simulink model "SimulinkController"  (R2016b)
settings: Solver=VariableStepAuto  StartTime=0.0  StopTime=40.0  RelTol=1e-3
undefined symbols (not defined in the file): K
settings Model: Creator=kwstas  LastModifiedBy=kwstas
settings SolverCC: MaxConsecutiveZCs=10000

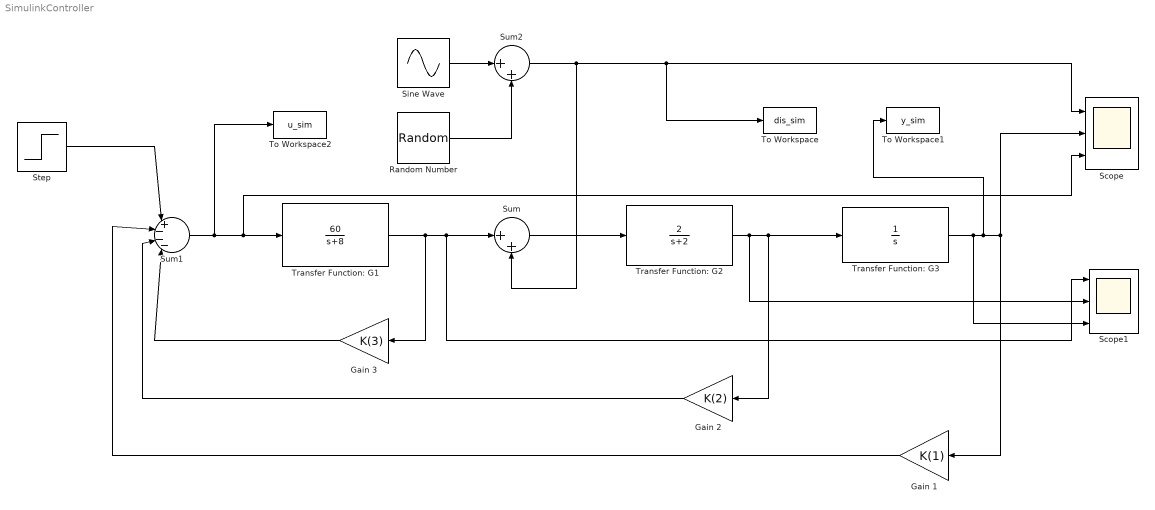
== system SimulinkController ==
  Gain 1 : Gain  Gain=K(1)
  "Gain 2 " : Gain  Gain=K(2)
  "Gain 3 " : Gain  Gain=K(3)
  Random Number : RandomNumber  Variance=5  SampleTime=0.1
  Scope : Scope  NumInputPorts=3
  Scope1 : Scope  NumInputPorts=3
  Sine Wave : Sin  Frequency=0.8  SampleTime=0
  Step : Step  Time=0  After=0  SampleTime=0
  Sum : Sum  Inputs=|++
  Sum1 : Sum  Inputs=|+---|
  Sum2 : Sum  Inputs=|++
  To Workspace : ToWorkspace  VariableName=dis_sim  SaveFormat=Timeseries  SampleTime=-1
  To Workspace1 : ToWorkspace  VariableName=y_sim  SaveFormat=Timeseries  SampleTime=-1
  To Workspace2 : ToWorkspace  VariableName=u_sim  SaveFormat=Timeseries  SampleTime=-1
  Transfer Function: G1 : TransferFcn  Numerator=[60]  Denominator=[1 8]
  "Transfer Function: G2 " : TransferFcn  Numerator=[2]  Denominator=[1 2]
  Transfer Function: G3 : TransferFcn  Denominator=[1 0]
  wires:
  Transfer Function: G1/1 -> "Gain 3 "/1, Scope1/1, Sum/1
  Sum/1 -> "Transfer Function: G2 "/1
  Sum1/1 -> To Workspace2/1, Scope/3, Transfer Function: G1/1
  "Transfer Function: G2 "/1 -> Scope1/2, "Gain 2 "/1, Transfer Function: G3/1
  Transfer Function: G3/1 -> Scope1/3, To Workspace1/1, Scope/2, Gain 1/1
  Gain 1/1 -> Sum1/2
  "Gain 2 "/1 -> Sum1/3
  "Gain 3 "/1 -> Sum1/4
  Step/1 -> Sum1/1
  Sum2/1 -> To Workspace/1, Scope/1, Sum/2
  Sine Wave/1 -> Sum2/1
  Random Number/1 -> Sum2/2
